simulink model "wecModel_Morrison_Heave_091514"  (R2014a)
settings: Solver=ode4  StartTime=0  StopTime=200  FixedStep=0.05  RelTol=1e-3
undefined symbols (not defined in the file): body, constraint, simu, waves, X, Y, Z
libraries: nesl_utility x18, vrlib x8, sm_lib x7, WECSim_Lib x2
(part 2 of 2)

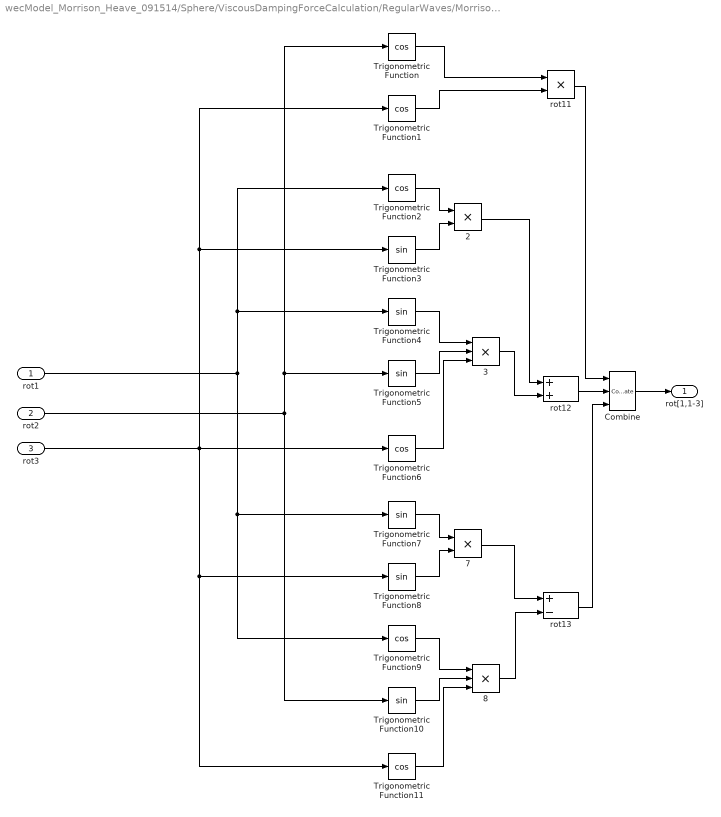
== system wecModel_Morrison_Heave_091514/Sphere/ViscousDampingForceCalculation/RegularWaves/MorrisonElements/Rotation1 ==
  rot1 : Inport
  rot2 : Inport  Port=2
  rot3 : Inport  Port=3
  2 : Product
  3 : Product  Inputs=3
  7 : Product
  8 : Product  Inputs=3
  Combine : Concatenate  NumInputs=3  Mode=Multidimensional array  ConcatenateDimension=2
  Trigonometric Function{,1..2,6,9,11} (6 alike) : Trigonometry  Operator=cos
  Trigonometric Function{3..5,7..8,10} (6 alike) : Trigonometry
  rot11 : Product
  rot12 : Sum
  rot13 : Sum  Inputs=+-
  rot[1,1-3] : Outport
  wires:
  Trigonometric Function/1 -> rot11/1
  Trigonometric Function1/1 -> rot11/2
  rot11/1 -> Combine/1
  Trigonometric Function2/1 -> 2/1
  Trigonometric Function3/1 -> 2/2
  Trigonometric Function4/1 -> 3/1
  Trigonometric Function5/1 -> 3/2
  Trigonometric Function6/1 -> 3/3
  2/1 -> rot12/1
  3/1 -> rot12/2
  rot12/1 -> Combine/2
  Combine/1 -> rot[1,1-3]/1
  rot2/1 -> Trigonometric Function/1, Trigonometric Function5/1, Trigonometric Function10/1
  rot3/1 -> Trigonometric Function1/1, Trigonometric Function3/1, Trigonometric Function6/1, Trigonometric Function11/1, Trigonometric Function8/1
  rot1/1 -> Trigonometric Function2/1, Trigonometric Function4/1, Trigonometric Function9/1, Trigonometric Function7/1
  Trigonometric Function7/1 -> 7/1
  Trigonometric Function8/1 -> 7/2
  Trigonometric Function9/1 -> 8/1
  Trigonometric Function10/1 -> 8/2
  Trigonometric Function11/1 -> 8/3
  7/1 -> rot13/1
  8/1 -> rot13/2
  rot13/1 -> Combine/3

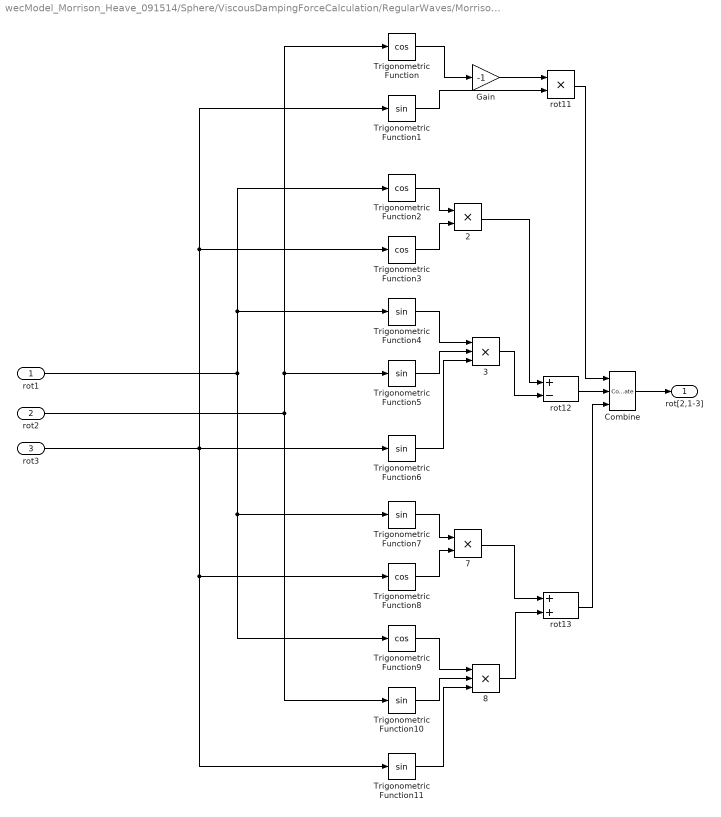
== system wecModel_Morrison_Heave_091514/Sphere/ViscousDampingForceCalculation/RegularWaves/MorrisonElements/Rotation2 ==
  rot1 : Inport
  rot2 : Inport  Port=2
  rot3 : Inport  Port=3
  2 : Product
  3 : Product  Inputs=3
  7 : Product
  8 : Product  Inputs=3
  Combine : Concatenate  NumInputs=3  Mode=Multidimensional array  ConcatenateDimension=2
  Gain : Gain  Gain=-1
  Trigonometric Function{,2..3,8..9} (5 alike) : Trigonometry  Operator=cos
  Trigonometric Function{1,4..7,10..11} (7 alike) : Trigonometry
  rot11 : Product
  rot12 : Sum  Inputs=+-
  rot13 : Sum
  rot[2,1-3] : Outport
  wires:
  Trigonometric Function/1 -> Gain/1
  Trigonometric Function1/1 -> rot11/2
  rot11/1 -> Combine/1
  Trigonometric Function2/1 -> 2/1
  Trigonometric Function3/1 -> 2/2
  Trigonometric Function4/1 -> 3/1
  Trigonometric Function5/1 -> 3/2
  Trigonometric Function6/1 -> 3/3
  2/1 -> rot12/1
  3/1 -> rot12/2
  rot12/1 -> Combine/2
  Combine/1 -> rot[2,1-3]/1
  rot2/1 -> Trigonometric Function/1, Trigonometric Function5/1, Trigonometric Function10/1
  rot3/1 -> Trigonometric Function1/1, Trigonometric Function3/1, Trigonometric Function6/1, Trigonometric Function11/1, Trigonometric Function8/1
  rot1/1 -> Trigonometric Function2/1, Trigonometric Function4/1, Trigonometric Function9/1, Trigonometric Function7/1
  Trigonometric Function7/1 -> 7/1
  Trigonometric Function8/1 -> 7/2
  Trigonometric Function9/1 -> 8/1
  Trigonometric Function10/1 -> 8/2
  Trigonometric Function11/1 -> 8/3
  7/1 -> rot13/1
  8/1 -> rot13/2
  rot13/1 -> Combine/3
  Gain/1 -> rot11/1

== system wecModel_Morrison_Heave_091514/Sphere/ViscousDampingForceCalculation/RegularWaves/MorrisonElements/Rotation3 ==
  rot1 : Inport
  rot2 : Inport  Port=2
  2 : Product
  7 : Product
  Combine : Concatenate  NumInputs=3  Mode=Multidimensional array  ConcatenateDimension=2
  Gain1 : Gain  Gain=-1
  TrigFun1 : Trigonometry
  TrigFun2 : Trigonometry
  TrigFun3 : Trigonometry  Operator=cos
  TrigFun4 : Trigonometry  Operator=cos
  TrigFun5 : Trigonometry  Operator=cos
  rot[3,1-3] : Outport
  wires:
  TrigFun1/1 -> Combine/1
  TrigFun3/1 -> 2/2
  2/1 -> Combine/2
  Combine/1 -> rot[3,1-3]/1
  rot2/1 -> TrigFun5/1, TrigFun3/1, TrigFun1/1
  TrigFun4/1 -> 7/1
  TrigFun5/1 -> 7/2
  rot1/1 -> TrigFun2/1, TrigFun4/1
  7/1 -> Combine/3
  TrigFun2/1 -> Gain1/1
  Gain1/1 -> 2/1

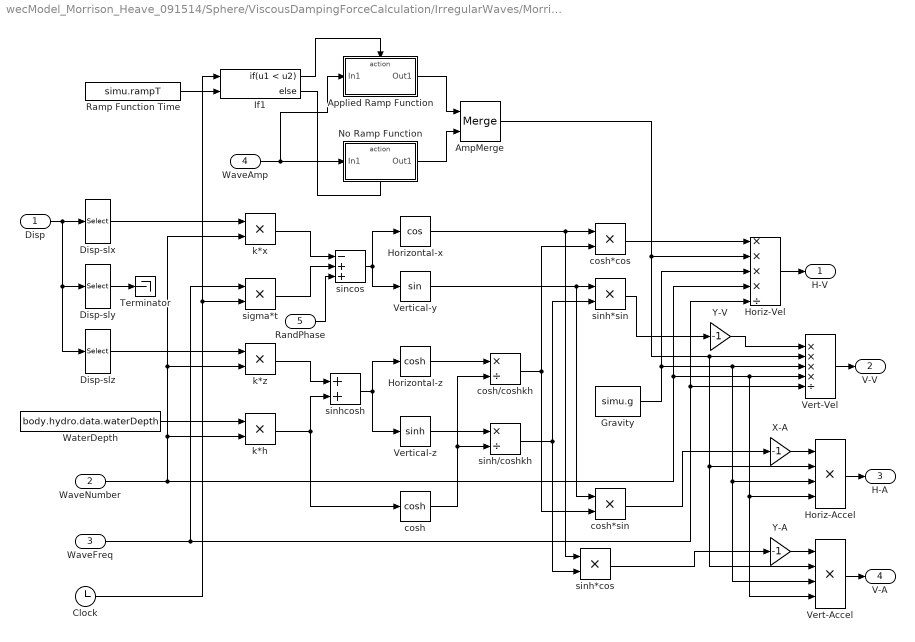
== system wecModel_Morrison_Heave_091514/Sphere/ViscousDampingForceCalculation/IrregularWaves/MorrisonElements/MorisonElementIrregular/OrbitalVelocity ==
  Disp : Inport
  WaveNumber : Inport  Port=2
  WaveFreq : Inport  Port=3
  WaveAmp : Inport  Port=4
  RandPhase : Inport  Port=5
  AmpMerge : Merge
  Applied Ramp Function : Subsystem  TreatAsAtomicUnit=on
  Clock : Clock
  Disp-slx : Selector  InputPortWidth=3  Indices=[1]
  Disp-sly : Selector  InputPortWidth=3  Indices=[2]
  Disp-slz : Selector  InputPortWidth=3  Indices=[3]
  Gravity : Constant  Value=simu.g
  Horiz-Accel : Product  Inputs=****
  Horiz-Vel : Product  Inputs=****/
  Horizontal-x : Trigonometry  Operator=cos
  Horizontal-z : Trigonometry  Operator=cosh
  If1 : If  NumInputs=2  IfExpression=u1 < u2
  No Ramp Function : Subsystem  TreatAsAtomicUnit=on
  Ramp Function Time : Constant  Value=simu.rampT
  Terminator : Terminator
  Vert-Accel : Product  Inputs=****
  Vert-Vel : Product  Inputs=****/
  Vertical-y : Trigonometry
  Vertical-z : Trigonometry  Operator=sinh
  WaterDepth : Constant  Value=body.hydro.data.waterDepth
  X-A : Gain  Gain=-1
  Y-A : Gain  Gain=-1
  Y-V : Gain  Gain=-1
  cosh : Trigonometry  Operator=cosh
  cosh*cos : Product  Inputs=**
  cosh*sin : Product  Inputs=**
  cosh/coshkh : Product  Inputs=*/
  k*h : Product
  k*x : Product
  k*z : Product
  sigma*t : Product
  sincos : Sum  Inputs=-++
  sinh*cos : Product  Inputs=**
  sinh*sin : Product  Inputs=**
  sinh/coshkh : Product  Inputs=*/
  sinhcosh : Sum
  H-V : Outport
  V-V : Outport  Port=2
  H-A : Outport  Port=3
  V-A : Outport  Port=4
  wires:
  Disp/1 -> Disp-slz/1, Disp-sly/1, Disp-slx/1
  Disp-slx/1 -> k*x/1
  WaveNumber/1 -> Vert-Vel/4, Vert-Accel/4, Horiz-Accel/4, Horiz-Vel/4, k*h/2, k*z/2, k*x/2
  WaveFreq/1 -> sigma*t/1, Horiz-Vel/5, Vert-Vel/5
  WaterDepth/1 -> k*h/1
  sigma*t/1 -> sincos/2
  k*x/1 -> sincos/1
  sincos/1 -> Vertical-y/1, Horizontal-x/1
  k*z/1 -> sinhcosh/1
  k*h/1 -> cosh/1, sinhcosh/2
  sinhcosh/1 -> Vertical-z/1, Horizontal-z/1
  Horizontal-z/1 -> cosh/coshkh/1
  cosh/1 -> sinh/coshkh/2, cosh/coshkh/2
  Vertical-z/1 -> sinh/coshkh/1
  Vertical-y/1 -> sinh*sin/1, cosh*sin/1
  sinh/coshkh/1 -> sinh*cos/2, sinh*sin/2
  Horizontal-x/1 -> cosh*cos/1, sinh*cos/1
  cosh/coshkh/1 -> cosh*cos/2, cosh*sin/2
  Disp-sly/1 -> Terminator/1
  cosh*cos/1 -> Horiz-Vel/1
  AmpMerge/1 -> Vert-Vel/2, Vert-Accel/2, Horiz-Accel/2, Horiz-Vel/2
  Gravity/1 -> Vert-Vel/3, Vert-Accel/3, Horiz-Accel/3, Horiz-Vel/3
  sinh*sin/1 -> Y-V/1
  Y-V/1 -> Vert-Vel/1
  X-A/1 -> Horiz-Accel/1
  Y-A/1 -> Vert-Accel/1
  Horiz-Vel/1 -> H-V/1
  Vert-Vel/1 -> V-V/1
  Horiz-Accel/1 -> H-A/1
  Vert-Accel/1 -> V-A/1
  cosh*sin/1 -> X-A/1
  sinh*cos/1 -> Y-A/1
  Ramp Function Time/1 -> If1/2
  If1/2 -> No Ramp Function/Action
  If1/1 -> Applied Ramp Function/Action
  Clock/1 -> If1/1, sigma*t/2
  WaveAmp/1 -> Applied Ramp Function/1(In1), No Ramp Function/1(In1)
  No Ramp Function/1(Out1) -> AmpMerge/2
  Applied Ramp Function/1(Out1) -> AmpMerge/1
  Disp-slz/1 -> k*z/1
  RandPhase/1 -> sincos/3

== system wecModel_Morrison_Heave_091514/Sphere/ViscousDampingForceCalculation/RegularWaves/MorrisonElements/OrbitalVelocity/Applied Ramp Function ==
  In1 : Inport
  Action Port : ActionPort
  Add : Sum
  Constant : Constant  Value=2
  Constant1 : Constant
  Divide : Product  Inputs=**/
  Sine Wave : Sin  Frequency=pi/simu.rampT  Phase=pi+pi/2  SampleTime=0
  Out1 : Outport
  wires:
  In1/1 -> Divide/1
  Divide/1 -> Out1/1
  Constant/1 -> Divide/3
  Constant1/1 -> Add/1
  Sine Wave/1 -> Add/2
  Add/1 -> Divide/2

== system wecModel_Morrison_Heave_091514/Sphere/ViscousDampingForceCalculation/RegularWaves/MorrisonElements/OrbitalVelocity/No Ramp Function ==
  In1 : Inport
  Action Port : ActionPort
  Out1 : Outport
  wires:
  In1/1 -> Out1/1

== system wecModel_Morrison_Heave_091514/Sphere/ViscousDampingForceCalculation/IrregularWaves/MorrisonElements/MorisonElementIrregular/OrbitalVelocity/Applied Ramp Function ==
  In1 : Inport
  Action Port : ActionPort
  Add : Sum
  Constant : Constant  Value=2
  Constant1 : Constant
  Divide : Product  Inputs=**/
  Sine Wave : Sin  Frequency=pi/simu.rampT  Phase=pi+pi/2  SampleTime=0
  Out1 : Outport
  wires:
  In1/1 -> Divide/1
  Divide/1 -> Out1/1
  Constant/1 -> Divide/3
  Constant1/1 -> Add/1
  Sine Wave/1 -> Add/2
  Add/1 -> Divide/2

== system wecModel_Morrison_Heave_091514/Sphere/ViscousDampingForceCalculation/IrregularWaves/MorrisonElements/MorisonElementIrregular/OrbitalVelocity/No Ramp Function ==
  In1 : Inport
  Action Port : ActionPort
  Out1 : Outport
  wires:
  In1/1 -> Out1/1

== matlab function wecModel_Morrison_Heave_091514/Sphere/Wave Radiation Forces Calculation/Fluid Memory ==
  data: check input; v input; F_FM output; ZeroVel input; IRKB input; CTTime input
function F_FM = ConvolutionalIntegral(check,v,ZeroVel,IRKB,CTTime)

%define persistent variables
persistent velocity;
persistent kkk

if check==10
    tmpT = zeros(6,1);
else
    if isempty(velocity)
       velocity = ZeroVel;
       kkk=0;
    else
       kkk=kkk+1;         
       velocity(:,1) = v(:);
       int2=kkk-floor((kkk)/5)*5;
       if int2<0.00000001
          velocity(:,2:end) = velocity(:,1:end-1);
       end
    end 
    
	%integrate
    tmpF = zeros(6,6);
    tmpT = zeros(6,1);
    for kd=1:6
        for kk=1:6
            tmpY=IRKB(:,kd,kk).*velocity(kk,:)';
            tmpF(kd,kk) = trapz(CTTime,tmpY);
        end
        tmpT(kd) = sum(tmpF(kd,1:6));
    end
end
F_FM=tmpT;
end

== matlab function wecModel_Morrison_Heave_091514/Sphere/Structure/Motion Sensor: Stucture Response/Angle ==
  data: Q input; E output
function E  = EulerAngle(Q)
%#codegen
E=zeros(3,1);
E(1) = atan2( (2*(Q(1)*Q(2)+Q(3)*Q(4))), (1-2* (Q(2)^2+Q(3)^2) ) );
E(2) = asin( 2* (Q(1)*Q(3) - Q(4)*Q(2)));
E(3) = atan2( (2*(Q(1)*Q(4)+Q(2)*Q(3))), (1-2* (Q(3)^2+Q(4)^2) ) );
